simulink model "Aufgabe5"  (R2016a)
settings: Solver=ode45  StartTime=0.0  StopTime=stop  MaxStep=1e-6  RelTol=1e-3
values from neighbouring files (symbols this model uses):
  f = 1e6    (= 1000000)    [Aufgabe5.m]
  fmod = 10e3    (= 10000)    [Aufgabe5.m]
  K0 = 2*pi*1e5    (= 628318.530718)    [Aufgabe5.m]
  tau1 = K0*Kd/w0^2    (= 3.18309886184e-06)    [Aufgabe5.m]
  tau2 = 2*zeta/w0-1/(K0*Kd)    (= 1.27323954474e-06)    [Aufgabe5.m]
libraries: commsynccomp2 x2, dsparch4 x1
settings Model: Creator=Martin Buchholz  LastModifiedBy=Marcel
settings DataIOCC: LimitDataPoints=on  SaveFormat=Array  SignalLoggingSaveFormat=ModelDataLogs
settings OptimizationCC: ExpressionDepthLimit=2147483647
settings DebuggingCC: UnderspecifiedInitializationDetection=Classic  MergeDetectMultiDrivingBlocksExec=none  SolverPrmCheckMsg=warning  FcnCallInpInsideContextMsg=UseLocalSettings  StateNameClashWarn=warning  StrictBusMsg=Warning
settings HardwareCC: ProdBitPerPointer=32  ProdLargestAtomicFloat=None  ProdIntDivRoundTo=Undefined  ProdEndianess=Unspecified  ProdWordSize=32  ProdHWDeviceType=32-bit Generic
settings ModelReferenceCC: PropagateSignalLabelsOutOfModel=off
settings GRTTargetCC: GeneratePreprocessorConditionals=Use local settings  CombineOutputUpdateFcns=off  GRTInterface=on
settings ConfigComp: CovModelRefEnable=Off

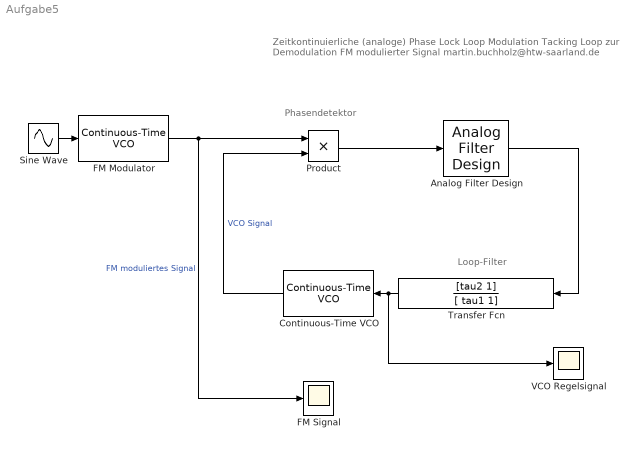
== system Aufgabe5 ==
  note: Zeitkontinuierliche (analoge) Phase Lock Loop
      |  Modulation Tacking Loop zur Demodulation FM modulierter Signal
      | martin.buchholz@htw-saarland.de
  note: Phasendetektor
  note: Loop-Filter
  Analog Filter Design : dsparch4/Analog Filter Design  method=Elliptic  filttype=Lowpass  N=4  Wlo=2*pi*f  Whi=80  Rp=1  Rs=40
  Continuous-Time VCO : commsynccomp2/Continuous-Time VCO  Ac=1  Fc=f  Kc=K0/(2*pi)  Ph=0
  FM Modulator : commsynccomp2/Continuous-Time VCO  Ac=1  Fc=f  Kc=df  Ph=0
  FM Signal : Scope
  Product : Product  RndMeth=Zero
  Sine Wave : Sin  Frequency=fmod  SampleTime=0
  Transfer Fcn : TransferFcn  Numerator=[tau2 1]  Denominator=[ tau1 1]
  VCO Regelsignal : Scope
  wires:
  FM Modulator/1 -> Product/1, FM Signal/1  "FM moduliertes Signal"
  Continuous-Time VCO/1 -> Product/2  "VCO Signal"
  Transfer Fcn/1 -> Continuous-Time VCO/1, VCO Regelsignal/1
  Product/1 -> Analog Filter Design/1
  Analog Filter Design/1 -> Transfer Fcn/1
  Sine Wave/1 -> FM Modulator/1
